simulink model "controller"  (R2022a)
settings: Solver=FixedStepDiscrete  StartTime=0.0  StopTime=inf  RelTol=1e-3  EnableMultiTasking=on
InitFcn:
  | run('busObjects.m')
model workspace (MAT data in the model file):
  omega = 8
  zeta = 0.05
libraries: aru_toolbox x1
settings Model: SimulationMode=external  Creator=Mechatronics  LastModifiedBy=Mechatronics
settings SolverCC: ConcurrentTasks=on  AlgebraicLoopSolver=TrustRegion  PositivePriorityOrder=on  InsertRTBMode=Never (minimum delay)
settings DataIOCC: SaveFormat=Array  SaveState=on  SignalLoggingName=logsOut
settings OptimizationCC: BlockReduction=off  BooleanDataType=off  OptimizeBlockIOStorage=off  BufferReuse=off  GlobalBufferReuse=off  ExpressionFolding=off  LocalBlockOutputs=off  InitFltsAndDblsToZero=on  OptimizeDataStoreBuffers=off  BusAssignmentInplaceUpdate=off
settings DebuggingCC: SaveWithParameterizedLinksMsg=none  UnderspecifiedInitializationDetection=Classic  MergeDetectMultiDrivingBlocksExec=none  CheckExecutionContextPreStartOutputMsg=on  SignalResolutionControl=TryResolveAllWithWarning  TasksWithSamePriorityMsg=none  UnconnectedInputMsg=warning  UnconnectedOutputMsg=warning  UnconnectedLineMsg=warning  SFUnexpectedBacktrackingDiag=warning  SFNoUnconditionalDefaultTransitionDiag=warning  SFExecutionAtInitializationDiag=none  SFMachineParentedDataDiag=warning  ArithmeticOperatorsInVariantConditions=warning
settings HardwareCC: ProdBitPerLong=64  ProdLongLongMode=on  ProdHWDeviceType=Intel->x86-64 (Linux 64)
settings ModelReferenceCC: PropagateSignalLabelsOutOfModel=off
settings SFSimCC: SimUseLocalCustomCode=off  SimTargetLang=C++
settings RTWCC: Description=Simulink Real-Time  SystemTargetFile=slrealtime.tlc  TemplateMakefile=slrealtime_default_tmf  RTWUseLocalCustomCode=off  Toolchain=Simulink Real-Time Toolchain  BuildConfiguration=Faster Runs  CodeExecutionProfiling=on  TargetLang=C++  DLArmComputeVersion=19.05
settings CodeAppCC: StateflowObjectComments=on
settings SimulinkRealTimeTargetCC: MATLABClassNameForMDSCustomization=Simulink.SoftwareTarget.GRTCustomization  UseGCCFastMath=on
settings ConfigComp: CovMetricSettings=dw  CovSaveCumulativeToWorkspaceVar=on  CovSaveSingleToWorkspaceVar=on  CovExternalEMLEnable=off  CovSFcnEnable=off

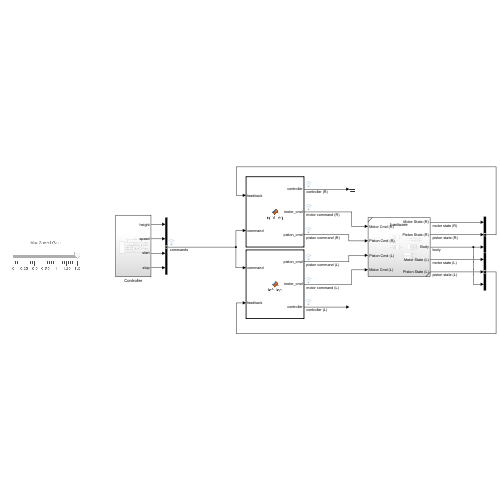
[thumbnail: Simulink's stored preview of the top-level diagram]
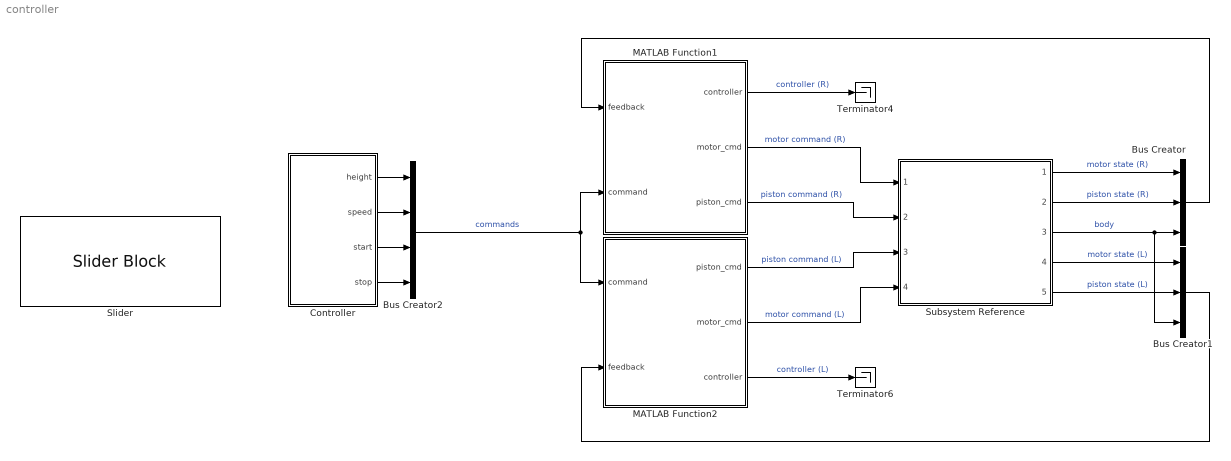
== system controller ==
  Bus Creator : BusCreator  Inputs=3  OutDataTypeStr=Bus: State  NonVirtualBus=on
      settings: InheritFromInputs=off
  Bus Creator1 : BusCreator  Inputs=3  OutDataTypeStr=Bus: State  NonVirtualBus=on
      settings: InheritFromInputs=off
  Bus Creator2 : BusCreator  Inputs=4  OutDataTypeStr=Bus: Command  NonVirtualBus=on
      settings: InheritFromInputs=off
  Controller : Subsystem
  MATLAB Function1 : MATLAB Function  TreatAsAtomicUnit=on  SystemSampleTime=0.001
  MATLAB Function2 : MATLAB Function  TreatAsAtomicUnit=on  SystemSampleTime=0.001
  Slider : SliderBlock  ScaleMax=1.5
  Subsystem Reference : Subsystem  ReferencedSubsystem=hardware
  Terminator4 : Terminator
  Terminator6 : Terminator
  wires:
  MATLAB Function1/3(piston_cmd) -> Subsystem Reference/2  "piston command (R)"
  MATLAB Function2/1(piston_cmd) -> Subsystem Reference/3  "piston command (L)"
  MATLAB Function1/2(motor_cmd) -> Subsystem Reference/1  "motor command (R)"
  MATLAB Function2/2(motor_cmd) -> Subsystem Reference/4  "motor command (L)"
  Subsystem Reference/4 -> Bus Creator1/1  "motor state (L)"
  Subsystem Reference/5 -> Bus Creator1/2  "piston state (L)"
  Subsystem Reference/3 -> Bus Creator1/3, Bus Creator/3  "body"
  Subsystem Reference/2 -> Bus Creator/2  "piston state (R)"
  Subsystem Reference/1 -> Bus Creator/1  "motor state (R)"
  Bus Creator/1 -> MATLAB Function1/1(feedback)
  Bus Creator1/1 -> MATLAB Function2/2(feedback)
  Bus Creator2/1 -> MATLAB Function2/1(command), MATLAB Function1/2(command)  "commands"
  Controller/2(speed) -> Bus Creator2/2
  MATLAB Function1/1(controller) -> Terminator4/1  "controller (R)"
  MATLAB Function2/3(controller) -> Terminator6/1  "controller (L)"
  Controller/1(height) -> Bus Creator2/1
  Controller/3(start) -> Bus Creator2/3
  Controller/4(stop) -> Bus Creator2/4

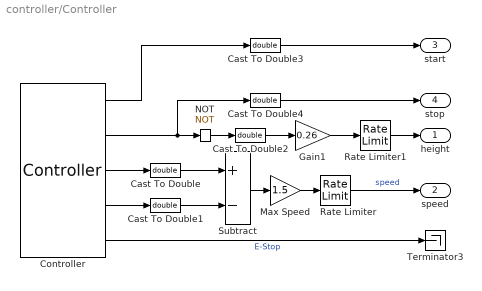
== system controller/Controller ==
  Cast To Double{,1..4} (5 alike) : DataTypeConversion  OutDataTypeStr=double  SaturateOnIntegerOverflow=off  RndMeth=Floor
  Controller : aru_toolbox/Controller
      link override "LVTTL digital input ": parInternalModuleId=1
      settings: SourceProductName=ARU Toolbox
  Gain1 : Gain  Gain=0.26
  Max Speed : Gain  Gain=1.5
  NOT : Logic  Operator=NOT  IconShape=distinctive  AllPortsSameDT=off  OutDataTypeStr=boolean
  Rate Limiter : RateLimiter  RisingSlewLimit=0.5  FallingSlewLimit=-0.5  SampleTimeMode=inherited
  Rate Limiter1 : RateLimiter  RisingSlewLimit=0.05  FallingSlewLimit=-0.05  SampleTimeMode=inherited  InitialCondition=0.26
  Subtract : Sum  Inputs=+-
  Terminator3 : Terminator
  height : Outport
  speed : Outport  Port=2
  start : Outport  Port=3
  stop : Outport  Port=4
  wires:
  Gain1/1 -> Rate Limiter1/1
  Rate Limiter/1 -> speed/1  "speed"
  Subtract/1 -> Max Speed/1
  Controller/5 -> Terminator3/1  "E-Stop"
  Controller/2 -> Cast To Double4/1, NOT/1
  Controller/3 -> Cast To Double/1
  Max Speed/1 -> Rate Limiter/1
  Controller/4 -> Cast To Double1/1
  Cast To Double/1 -> Subtract/1
  Cast To Double1/1 -> Subtract/2
  Controller/1 -> Cast To Double3/1
  Rate Limiter1/1 -> height/1
  Cast To Double3/1 -> start/1
  NOT/1 -> Cast To Double2/1
  Cast To Double2/1 -> Gain1/1
  Cast To Double4/1 -> stop/1

== matlab function controller/MATLAB Function2 ==
  data: command input Bus: Command; feedback input Bus: State; piston_cmd output Bus: PistonCmd; motor_cmd output Bus: MotorCmd; controller output Bus: Controller
function [piston_cmd, motor_cmd, controller] = left_leg(command, feedback) %#codegen

% initialisation
hip.y = 0; hip.dy = 0; hip.y_min = 0; hip.y_max = 0;
foot.y = 0; foot.height = 0; foot.contact = false; foot.radius = 20e-3;

% constants
contact_threshold = 1e-2; % m foot radius
contact_acceleration_threshold = -100; % m/s^2
retract_duration = 17; % 17ms
hip.amplitude = 0.01;
hip.y_min = command.height - 0.5*hip.amplitude;
hip.y_max = command.height + 0.5*hip.amplitude;

motor = feedback.Motor;
piston = feedback.Piston;
body = feedback.Body;

% kinematics
[r,dr,phi,~] = virtural_leg_b(piston.v, body.dr, motor.w, piston.p, body.r, motor.q);
[~, ~ ,hip.y, hip.dy] = hip_pos_b(body.dr, body.dx, body.dy, body.r, body.x, body.y);
[~,foot.y] = foot_pos_b(piston.p, body.r, motor.q, body.x, body.y);

persistent state
persistent retract_timer
persistent ground_offset
persistent Ts
if isempty(state)
    state = States.Rest;
end
if isempty(retract_timer)
    retract_timer = 0;
end
if isempty(ground_offset)
    ground_offset = 0;
end
if isempty(Ts)
    Ts = 0;
end

% contact detection
foot.height = foot.y + ground_offset;
if foot.height > contact_threshold
    foot.contact = false;
else
    foot.contact = true;
end

% state transitions
switch(state)
    case States.Rest
        if (body.r > 0.1) && (command.start) % wait until right leg has pushed off a bit
            state = States.Stance;
            ground_offset = -foot.y;
        end
    case States.Flight
        if ((hip.y + ground_offset) < ((2.5*hip.dy*hip.dy)/(2*50) + hip.y_min)) && (hip.dy < 0)
            state = States.Loading;
        elseif (hip.y_min < 0.17) && (command.stop)
            state = States.Rest;
        end
    case States.Loading
        if (piston.a < contact_acceleration_threshold) || (foot.contact)
            Ts = 0;
            state = States.Stance;
        end
    case States.Stance
        if hip.dy > 0
            if (hip.y + ground_offset) > ((hip.dy*hip.dy)/(-2*9.81) + hip.y_max)
                retract_timer = 0;
                ground_offset = -foot.y; % update ground offset
                state = States.Unloading;
            end
        end
    case States.Unloading
        if ~foot.contact
            state = States.Flight;
        end
end


% control piston
switch(state)
    case {States.Loading, States.Stance}
        piston_cmd.ue = 1;
        piston_cmd.ur = 0;
    case States.Unloading
        piston_cmd.ue = 0;
        if retract_timer < retract_duration
            piston_cmd.ur = 1;
        else
            piston_cmd.ur = 0;
        end
        retract_timer = retract_timer + 1;
    otherwise
        piston_cmd.ue = 0;
        piston_cmd.ur = 0;
end

% stance timer
switch(state)
    case {States.Stance, States.Unloading}
        Ts = Ts + 0.001;
end

% control motor
switch(state)
    case {States.Stance, States.Unloading, States.Loading}
        phi_d = -pi/2;
        dphi_d = (dr*cos(phi) + command.speed)/(r*sin(phi));
        Kp = 0;
        Kd = 4;
    case {States.Flight}
        foot_offset = (body.dx*(0.1))/(2*r);
        foot_offset = max(min(foot_offset,1),-1);
        phi_d = -pi/2 + asin(foot_offset);
        dphi_d = 0;
        Kp = 100; % 80
        Kd = 4;
    otherwise
        phi_d = -pi/2;
        dphi_d = 0;
        Kp = 50;
        Kd = 4;
end
 
[theta_m_des,dtheta_m_des] = phi_tracking_b(piston.v, dphi_d, body.dr, piston.p, phi_d, body.r);
% bound motor angle to not break pneumatics
theta_m_des =  min(theta_m_des, 0);

motor_cmd.q = theta_m_des;
motor_cmd.w = dtheta_m_des;
motor_cmd.Kp = Kp;
motor_cmd.Kd = Kd;
motor_cmd.tff = 0;

controller.state = state;
controller.Ts = Ts;
 
end

== matlab function controller/MATLAB Function1 ==
  data: feedback input Bus: State; controller output Bus: Controller; motor_cmd output Bus: MotorCmd; piston_cmd output Bus: PistonCmd; command input Bus: Command
function [controller, motor_cmd, piston_cmd] = right_leg(feedback, command) %#codegen

% initialisation
hip.y = 0; hip.dy = 0; hip.y_min = 0; hip.y_max = 0;
foot.y = 0; foot.height = 0; foot.contact = false; foot.radius = 20e-3;

motor = feedback.Motor;
piston = feedback.Piston;
body = feedback.Body;

% kinematics
[r,dr,phi,~] = virtural_leg_f(piston.v, body.dr, motor.w, piston.p, body.r, motor.q);
[~, ~ ,hip.y, hip.dy] = hip_pos_f(body.dr, body.dx, body.dy, body.r, body.x, body.y);
[~,foot.y] = foot_pos_f(piston.p, body.r, motor.q, body.x, body.y);

% constants
contact_threshold = 1e-2; % m relies on ground being flat
contact_acceleration_threshold = -100; % m/s^2
retract_duration = 17; % 17ms
hip.amplitude = 0.01;
hip.y_min = command.height - 0.5*hip.amplitude;
hip.y_max = command.height + 0.5*hip.amplitude;

persistent state
persistent retract_timer
persistent ground_offset
persistent Ts
if isempty(state)
    state = States.Rest;
end
if isempty(retract_timer)
    retract_timer = 0;
end
if isempty(ground_offset)
    ground_offset = 0;
end
if isempty(Ts)
    Ts = 0;
end
 
% contact detection
foot.height = foot.y + ground_offset;
if foot.height > contact_threshold
    foot.contact = false;
else
    foot.contact = true;
end
 
% state transitions
switch(state)
    case States.Rest
        if command.start
            state = States.Stance;
            ground_offset = -foot.y;
        end
    case States.Flight
        if ((hip.y + ground_offset) < ((2.5*hip.dy*hip.dy)/(2*50) + hip.y_min)) && (hip.dy < 0)
            state = States.Loading;
        elseif (hip.y_min < 0.17) && (command.stop)
            state = States.Rest;
        end
    case States.Loading
        if (piston.a < contact_acceleration_threshold) || (foot.contact)
            Ts = 0;
            state = States.Stance;
        end
    case States.Stance
        if hip.dy > 0
            if (hip.y + ground_offset) > ((hip.dy*hip.dy)/(-2*9.81) + hip.y_max)
                retract_timer = 0;
                ground_offset = -foot.y; % update ground offset
                state = States.Unloading;
            end
        end
    case States.Unloading
        if ~foot.contact
            state = States.Flight;
        end
end
 
 
% control piston
switch(state)
    case {States.Loading, States.Stance}
        piston_cmd.ue = 1;
        piston_cmd.ur = 0;
    case States.Unloading
        piston_cmd.ue = 0;
        if retract_timer < retract_duration
            piston_cmd.ur = 1;
        else
            piston_cmd.ur = 0;
        end
        retract_timer = retract_timer + 1;
    otherwise
        piston_cmd.ue = 0;
        piston_cmd.ur = 0;
end

% stance timer
switch(state)
    case {States.Stance, States.Unloading}
        Ts = Ts + 0.001;
end
 
% control motor
switch(state)
    case {States.Stance, States.Unloading, States.Loading}
        phi_d = -pi/2;
        dphi_d = (dr*cos(phi) + command.speed)/(r*sin(phi));
        Kp = 0;
        Kd = 4;
    case {States.Flight}
        foot_offset = (body.dx*(0.1))/(2*r);
        foot_offset = max(min(foot_offset,1),-1);
        phi_d = -pi/2 + asin(foot_offset);
        dphi_d = 0;
        Kp = 100;
        Kd = 4;
    otherwise
        phi_d = -pi/2;
        dphi_d = 0;
        Kp = 50;
        Kd = 4;
end

[theta_m_des, dtheta_m_des] = phi_tracking_f(piston.v, dphi_d, body.dr, piston.p, phi_d, body.r);
% bound motor angle to not break pneumatics
theta_m_des = max(-pi, theta_m_des);

motor_cmd.q = theta_m_des;
motor_cmd.w = dtheta_m_des;
motor_cmd.Kp = Kp;
motor_cmd.Kd = Kd;
motor_cmd.tff = 0;

controller.state = state;
controller.Ts = Ts;
 
end
